simulink model "lyapanov"  (R2022b)
settings: Solver=VariableStepAuto  StartTime=0.0  StopTime=6000  RelTol=1e-4
values from neighbouring files (symbols this model uses):
  den_real = [1, (tau1 + tau2 + R2) / (tau1*tau2), 1/ (tau1*tau2)]    [SIMULATION_CODE.m]
  num_real = [R2/(tau1*tau2)]    [SIMULATION_CODE.m]
undefined symbols (not defined in the file or in its folder): den_des, num_des
libraries: dspsrcs4 x1
settings Model: Creator=mahdi  LastModifiedBy=user
settings DebuggingCC: UnconnectedInputMsg=warning  UnconnectedOutputMsg=warning  UnconnectedLineMsg=warning
settings ModelReferenceCC: EnableRefExpFcnMdlSchedulingChecks=on
settings RTWCC: DLArmComputeVersion=19.05

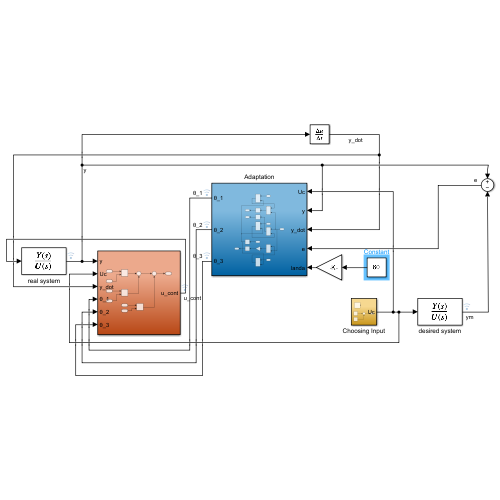
[thumbnail: Simulink's stored preview of the top-level diagram]
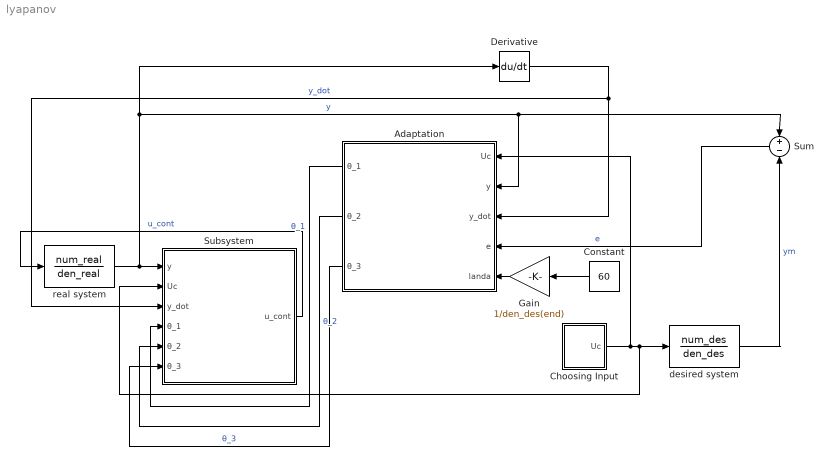
== system lyapanov ==
  Adaptation : Subsystem
  Choosing Input : Subsystem
  Constant : Constant  Value=60
  Derivative : Derivative
  Gain : Gain  Gain=1/den_des(end)
  Subsystem : Subsystem
  Sum : Sum  Inputs=+|-
  desired system : TransferFcn  Numerator=num_des  Denominator=den_des
  real system : TransferFcn  Numerator=num_real  Denominator=den_real
  wires:
  Gain/1 -> Adaptation/5(landa)
  Adaptation/1(θ_1) -> Subsystem/4(θ_1)  "θ_1"
  real system/1 -> Adaptation/2(y), Sum/1, Derivative/1, Subsystem/1(y)  "y"
  Subsystem/1(u_cont) -> real system/1  "u_cont"
  Adaptation/3(θ_3) -> Subsystem/6(θ_3)  "θ_3"
  Adaptation/2(θ_2) -> Subsystem/5(θ_2)  "θ_2"
  Derivative/1 -> Subsystem/3(y_dot), Adaptation/3(y_dot)  "y_dot"
  Choosing Input/1(Uc) -> Subsystem/2(Uc), desired system/1, Adaptation/1(Uc)
  Constant/1 -> Gain/1
  desired system/1 -> Sum/2  "ym"
  Sum/1 -> Adaptation/4(e)  "e"

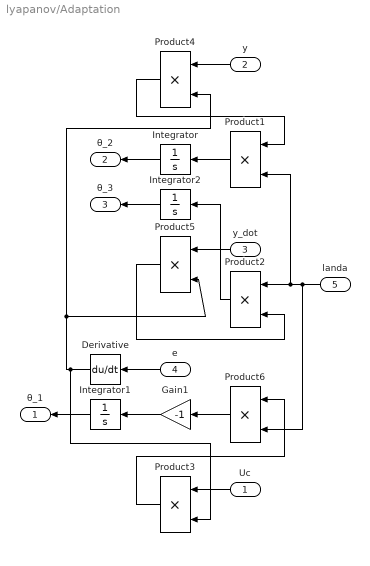
== system lyapanov/Adaptation ==
  Uc : Inport
  y : Inport  Port=2
  y_dot : Inport  Port=3
  e : Inport  Port=4
  landa : Inport  Port=5
  Derivative : Derivative
  Gain1 : Gain  Gain=-1
  Integrator : Integrator
  Integrator1 : Integrator
  Integrator2 : Integrator
  Product{1..6} (6 alike) : Product
  θ_1 : Outport
  θ_2 : Outport  Port=2
  θ_3 : Outport  Port=3
  wires:
  Product3/1 -> Product6/1
  Gain1/1 -> Integrator1/1
  e/1 -> Derivative/1
  Product5/1 -> Product2/2
  Product1/1 -> Integrator/1
  Integrator/1 -> θ_2/1
  Integrator1/1 -> θ_1/1
  Product4/1 -> Product1/1
  Derivative/1 -> Product5/2, Product4/2, Product3/2
  Integrator2/1 -> θ_3/1
  y/1 -> Product4/1
  y_dot/1 -> Product5/1
  Product2/1 -> Integrator2/1
  Product6/1 -> Gain1/1
  Uc/1 -> Product3/1
  landa/1 -> Product2/1, Product1/2, Product6/2

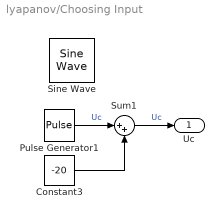
== system lyapanov/Choosing Input ==
  Constant3 : Constant  Value=-20
  Pulse Generator1 : DiscretePulseGenerator  PulseType=Time based  Amplitude=40  Period=3000  PulseWidth=50
  Sine Wave : dspsrcs4/Sine Wave  Amplitude=5  Frequency=0.001  Phase=0  SampleMode=Continuous  OutComplex=Real  CompMethod=Trigonometric fcn  TableSize=Speed  SampleTime=0  SamplesPerFrame=1  ResetState=Restart at time zero  OutputFrames=off  dataType=double  wordLen=16  udDataType=sfix(16)  fracBitsMode=Best precision  numFracBits=15  OutDataTypeStr=double  LastOutDataTypeStr=double
  Sum1 : Sum  Inputs=|++
  Uc : Outport
  wires:
  Pulse Generator1/1 -> Sum1/1  "Uc"
  Constant3/1 -> Sum1/2
  Sum1/1 -> Uc/1  "Uc"

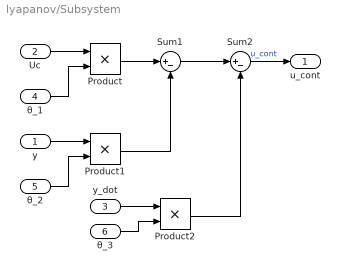
== system lyapanov/Subsystem ==
  y : Inport
  Uc : Inport  Port=2
  y_dot : Inport  Port=3
  θ_1 : Inport  Port=4
  θ_2 : Inport  Port=5
  θ_3 : Inport  Port=6
  Product : Product
  Product1 : Product
  Product2 : Product
  Sum1 : Sum  Inputs=|+-
  Sum2 : Sum  Inputs=|+-
  u_cont : Outport
  wires:
  θ_3/1 -> Product2/2
  y_dot/1 -> Product2/1
  θ_1/1 -> Product/2
  Product1/1 -> Sum1/2
  Sum1/1 -> Sum2/1
  Uc/1 -> Product/1
  Product/1 -> Sum1/1
  θ_2/1 -> Product1/2
  y/1 -> Product1/1
  Product2/1 -> Sum2/2
  Sum2/1 -> u_cont/1  "u_cont"
